simulink model "ARDroneBaseSim"  (R2013b)
settings: Solver=ode1  StartTime=0.0  StopTime=100  FixedStep=simDT  RelTol=1e-3
libraries: ARBlocks x1
settings Model: Creator=Paul Freeman  LastModifiedBy=david
settings DataIOCC: LimitDataPoints=off  SignalLoggingSaveFormat=ModelDataLogs  SaveOutput=off  SignalLogging=off
settings OptimizationCC: ExpressionDepthLimit=2147483647
settings DebuggingCC: MultiTaskDSMMsg=warning  MultiTaskCondExecSysMsg=none  FcnCallInpInsideContextMsg=UseLocalSettings  StateNameClashWarn=warning
settings HardwareCC: ProdLargestAtomicInteger=Long  ProdLargestAtomicFloat=Double  ProdIntDivRoundTo=Zero  ProdEndianess=BigEndian  ProdHWDeviceType=Freescale->32-bit PowerPC
settings SFSimCC: SimParseCustomCode=off
settings RTWCC: IncludeERTFirstTime=on
settings GRTTargetCC: CombineOutputUpdateFcns=off  GRTInterface=on

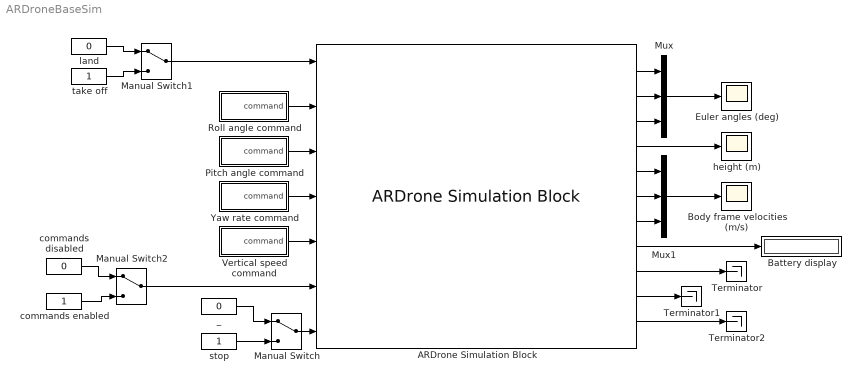
== system ARDroneBaseSim ==
  ARDrone Simulation Block : ARBlocks/ARDrone Simulation Block
  Battery display : Display
  Body frame velocities (m/s) : Scope
      settings: YMin=-22.5  YMax=22.5  SaveName=ScopeData2  MaxDataPoints=500000
  Euler angles (deg) : Scope
      settings: YMin=-22.5  YMax=22.5  MaxDataPoints=500000
  Manual Switch : ManualSwitch
  Manual Switch1 : ManualSwitch
  Manual Switch2 : ManualSwitch
  Mux : Mux  Inputs=3
  Mux1 : Mux  Inputs=3
  Pitch angle command : Subsystem
  Roll angle command : Subsystem
  Terminator : Terminator
  Terminator1 : Terminator
  Terminator2 : Terminator
  Vertical speed command : Subsystem
  Yaw rate command : Subsystem
  _ : Constant  Value=0
  commands disabled : Constant  Value=0
  commands enabled : Constant
  height (m) : Scope
      settings: YMin=-22.5  YMax=22.5  MaxDataPoints=500000
  land : Constant  Value=0
  stop : Constant
  take off : Constant
  wires:
  _/1 -> Manual Switch/1
  stop/1 -> Manual Switch/2
  land/1 -> Manual Switch1/1
  take off/1 -> Manual Switch1/2
  commands disabled/1 -> Manual Switch2/1
  commands enabled/1 -> Manual Switch2/2
  Manual Switch1/1 -> ARDrone Simulation Block/1
  Manual Switch2/1 -> ARDrone Simulation Block/6
  Manual Switch/1 -> ARDrone Simulation Block/7
  ARDrone Simulation Block/1 -> Mux/1
  ARDrone Simulation Block/2 -> Mux/2
  ARDrone Simulation Block/5 -> Mux1/1
  ARDrone Simulation Block/6 -> Mux1/2
  ARDrone Simulation Block/7 -> Mux1/3
  ARDrone Simulation Block/8 -> Battery display/1
  ARDrone Simulation Block/4 -> height (m)/1
  Mux1/1 -> Body frame velocities (m/s)/1
  ARDrone Simulation Block/3 -> Mux/3
  ARDrone Simulation Block/9 -> Terminator/1
  ARDrone Simulation Block/10 -> Terminator1/1
  ARDrone Simulation Block/11 -> Terminator2/1
  Mux/1 -> Euler angles (deg)/1
  Roll angle command/1(command) -> ARDrone Simulation Block/2
  Pitch angle command/1(command) -> ARDrone Simulation Block/3
  Yaw rate command/1(command) -> ARDrone Simulation Block/4
  Vertical speed command/1(command) -> ARDrone Simulation Block/5

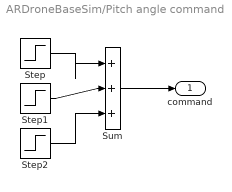
== system ARDroneBaseSim/Pitch angle command ==
  Step : Step  Time=14  SampleTime=0
  Step1 : Step  Time=18  After=-2  SampleTime=0
  Step2 : Step  Time=22  SampleTime=0
  Sum : Sum  Inputs=|+++
  command : Outport
  wires:
  Step1/1 -> Sum/2
  Step/1 -> Sum/1
  Step2/1 -> Sum/3
  Sum/1 -> command/1

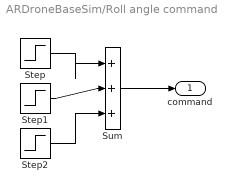
== system ARDroneBaseSim/Roll angle command ==
  Step : Step  Time=2  SampleTime=0
  Step1 : Step  Time=6  After=-2  SampleTime=0
  Step2 : Step  Time=10  SampleTime=0
  Sum : Sum  Inputs=|+++
  command : Outport
  wires:
  Step1/1 -> Sum/2
  Step/1 -> Sum/1
  Step2/1 -> Sum/3
  Sum/1 -> command/1

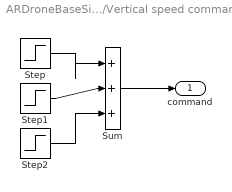
== system ARDroneBaseSim/Vertical speed command ==
  Step : Step  Time=34  SampleTime=0
  Step1 : Step  Time=36  After=-2  SampleTime=0
  Step2 : Step  Time=38  SampleTime=0
  Sum : Sum  Inputs=|+++
  command : Outport
  wires:
  Step1/1 -> Sum/2
  Step/1 -> Sum/1
  Step2/1 -> Sum/3
  Sum/1 -> command/1

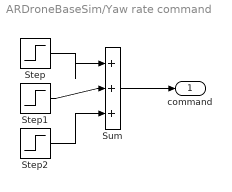
== system ARDroneBaseSim/Yaw rate command ==
  Step : Step  Time=26  SampleTime=0
  Step1 : Step  Time=28  After=-2  SampleTime=0
  Step2 : Step  Time=30  SampleTime=0
  Sum : Sum  Inputs=|+++
  command : Outport
  wires:
  Step1/1 -> Sum/2
  Step/1 -> Sum/1
  Step2/1 -> Sum/3
  Sum/1 -> command/1
